simulink model "pid_Modelo"  (R2021b)
settings: Solver=VariableStepAuto  StartTime=0.0  StopTime=1200  RelTol=1e-3
undefined symbols (not defined in the file or in its folder): magnitude, sigbuilder_block
libraries: slpidlib x1
settings Model: Creator=diego  LastModifiedBy=diego
settings SolverCC: AlgebraicLoopSolver=TrustRegion
settings DataIOCC: SaveOutput=off  SaveTime=off  ReturnWorkspaceOutputs=off
settings DebuggingCC: SFMachineParentedDataDiag=warning

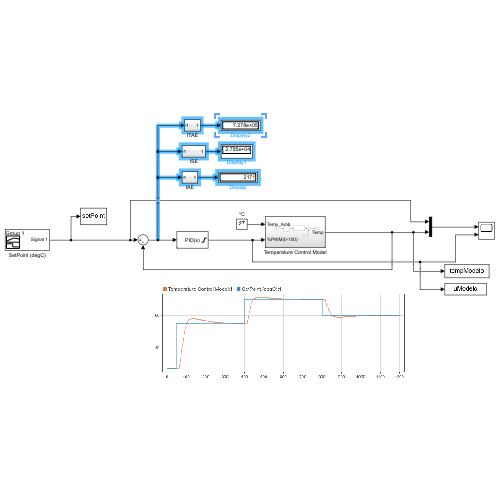
[thumbnail: Simulink's stored preview of the top-level diagram]
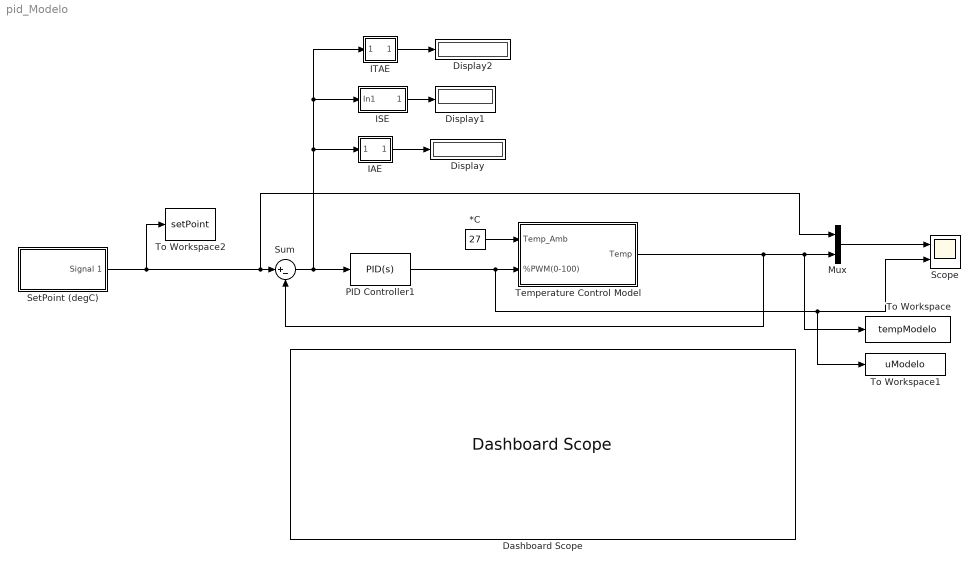
== system pid_Modelo ==
  *C : Constant  Value=27
  Dashboard Scope : DashboardScope  Ymin=23  Ymax=90
  Display : Display
  Display1 : Display
  Display2 : Display
  IAE : Subsystem
  ISE : Subsystem
  ITAE : Subsystem
  Mux : Mux  Inputs=2
  PID Controller1 : slpidlib/PID Controller  Controller=PID  Form=Parallel  TimeDomain=Continuous-time  UseExternalTs=off  SampleTime=-1  IntegratorMethod=Forward Euler  FilterMethod=Forward Euler  ControllerParametersSource=internal  P=3.58266232285661  I=0.0448736690379743  D=10.3284593159219  UseFilter=on  N=0.0959425813529886  TunerSelectOption=Transfer Function Based (PID Tuner App)  InitialConditionSource=internal  InitialConditionForIntegrator=0  InitialConditionForFilter=0  DifferentiatorICPrevScaledInput=0  ExternalReset=none  TrackingMode=off  Kt=1  LimitOutput=on  SatLimitsSource=internal  UpperSaturationLimit=100  LowerSaturationLimit=0  LinearizeAsGain=on  AntiWindupMode=none  Kb=1  POutMin=[]  POutMax=[]  IOutMin=[]  IOutMax=[]  DOutMin=[]  DOutMax=[]  NOutMin=[]  NOutMax=[]  SumOutMin=[]  SumOutMax=[]  SaturationOutMin=[]  SaturationOutMax=[]  PParamMin=[]  PParamMax=[]  IParamMin=[]  IParamMax=[]  DParamMin=[]  DParamMax=[]  NParamMin=[]  NParamMax=[]  KbParamMin=[]  KbParamMax=[]  KtParamMin=[]  KtParamMax=[]  KbOutMin=[]  KbOutMax=[]  KtOutMin=[]  KtOutMax=[]  IntegratorOutMin=[]  IntegratorOutMax=[]  FilterOutMin=[]  FilterOutMax=[]  SumI1OutMin=[]  SumI1OutMax=[]  SumI2OutMin=[]  SumI2OutMax=[]  SumI3OutMin=[]  SumI3OutMax=[]  SumI4OutMin=[]  SumI4OutMax=[]  SumDOutMin=[]  SumDOutMax=[]  DifferentiatorOutMin=[]  DifferentiatorOutMax=[]  FilterDiffOutCoefMin=[]  FilterDiffOutCoefMax=[]  ReciprocalOutMin=[]  ReciprocalOutMax=[]  SumDenOutMin=[]  SumDenOutMax=[]  SumNumOutMin=[]  SumNumOutMax=[]  DivideOutMin=[]  DivideOutMax=[]  UdiffTsProdOutMin=[]  UdiffTsProdOutMax=[]  NTsProdOutMin=[]  NTsProdOutMax=[]  UintegralTsProdOutMin=[]  UintegralTsProdOutMax=[]  UngainTsProdOutMin=[]  UngainTsProdOutMax=[]  IntegratorContinuousStateAttributes=''  IntegratorStateMustResolveToSignalObject=off  IntegratorRTWStateStorageClass=Auto  FilterContinuousStateAttributes=''  FilterStateMustResolveToSignalObject=off  FilterRTWStateStorageClass=Auto  ParallelPVariant=InternalParameters  IdealPVariant=Disabled  IVariant=InternalParameters  DVariant=InternalParameters  IntegratorVariant=Continuous  SatVariant=Enabled  AWVariant=Passthrough  PCopyVariant=Disabled  TRVariant=Disabled  FdbkBlocksVariant=Forward  IdealPFdbkVariant=Disabled  SatFdbkVariant=Disabled  DerivativeFilterVariant=ContFilter  NVariant=InternalParameters  NCopyVariant=Disabled  FilterICVariant=InternalICsFilter  IntegratorICVariant=InternalICs  ExternalResetVariant=Disabled  TRSumVariant=Passthrough  SumFdbkVariant=Disabled  SumVariant=Sum_PID  TsampFilterVariant=InternalTs  TsampNgainVariant=Passthrough  TsampIntegralVariant=Passthrough  ExternalSaturationOutDataTypeStr=Inherit: Same as second input
  Scope : Scope  NumInputPorts=2
  SetPoint (degC) : Subsystem  Tag=STV Subsys  LoadFcn=sigbuilder_block('load');  StartFcn=sigbuilder_block('start');  StopFcn=sigbuilder_block('stop');  ClipboardFcn=sigbuilder_block('clipboard');  mask(Sigbuilder block){tuvar=[0:10]}
      mask help: Simulink:masks:SigbuilderBlock_MD
      mask init:
      | if ~strcmp(get_param(bdroot(gcbh),'SimulationStatus'),'stopped') tuvar = sigbuilder_block('maskInit'); end
      settings: CopyFcn=sigbuilder_block('copy');  DeleteFcn=sigbuilder_block('delete');  ModelCloseFcn=sigbuilder_block('modelClose');  PreSaveFcn=sigbuilder_block('preSave');  PauseFcn=sigbuilder_block('pause');  ContinueFcn=sigbuilder_block('continue');  NameChangeFcn=sigbuilder_block('namechange');  OpenFcn=sigbuilder_block('open',[53.4 0 1093.2 552.6 ]);  CloseFcn=sigbuilder_block('close');
      mask Display: plot(0, 0, 100, 100,[2, 2, 32, 32, 2], [68, 8, 8, 68, 68],[32, 2], [38, 38], [32, 19, 2],[53, 60, 44], [32, 17, 17, 2],[16, 16, 31, 31]);txt = getActiveGroup(gcbh);text(2, 100, txt,'verticalAlignment', 'top');
  Sum : Sum  Inputs=|+-
  Temperature Control Model : Subsystem
  To Workspace : ToWorkspace  VariableName=tempModelo  SampleTime=1
      settings: Save2DSignal=2-D array (concatenate along first dimension)
  To Workspace1 : ToWorkspace  VariableName=uModelo  SampleTime=1
      settings: Save2DSignal=2-D array (concatenate along first dimension)
  To Workspace2 : ToWorkspace  VariableName=setPoint  SampleTime=1
      settings: Save2DSignal=2-D array (concatenate along first dimension)
  wires:
  SetPoint (degC)/1(Signal 1) -> To Workspace2/1, Mux/1, Sum/1
  Sum/1 -> ITAE/1(In1), ISE/1(In1), IAE/1(In1), PID Controller1/1
  *C/1 -> Temperature Control Model/1(Temp_Amb)
  PID Controller1/1 -> To Workspace1/1, Scope/2, Temperature Control Model/2(%PWM(0-100))
  Mux/1 -> Scope/1
  Temperature Control Model/1(Temp) -> Sum/2, To Workspace/1, Mux/2
  IAE/1(Out1) -> Display/1
  ITAE/1(Out1) -> Display2/1
  ISE/1(Out1) -> Display1/1

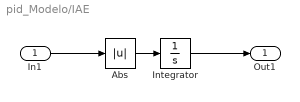
== system pid_Modelo/IAE ==
  In1 : Inport
  Abs : Abs
  Integrator : Integrator
  Out1 : Outport
  wires:
  Abs/1 -> Integrator/1
  In1/1 -> Abs/1
  Integrator/1 -> Out1/1

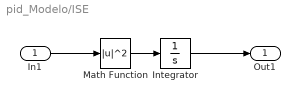
== system pid_Modelo/ISE ==
  In1 : Inport
  Integrator : Integrator
  Math Function : Math  Operator=magnitude^2  SaturateOnIntegerOverflow=on
  Out1 : Outport
  wires:
  Integrator/1 -> Out1/1
  In1/1 -> Math Function/1
  Math Function/1 -> Integrator/1

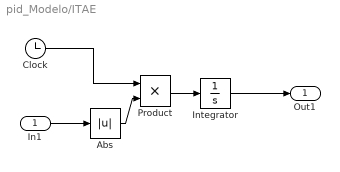
== system pid_Modelo/ITAE ==
  In1 : Inport
  Abs : Abs
  Clock : Clock
  Integrator : Integrator
  Product : Product
  Out1 : Outport
  wires:
  Integrator/1 -> Out1/1
  Product/1 -> Integrator/1
  In1/1 -> Abs/1
  Clock/1 -> Product/1
  Abs/1 -> Product/2

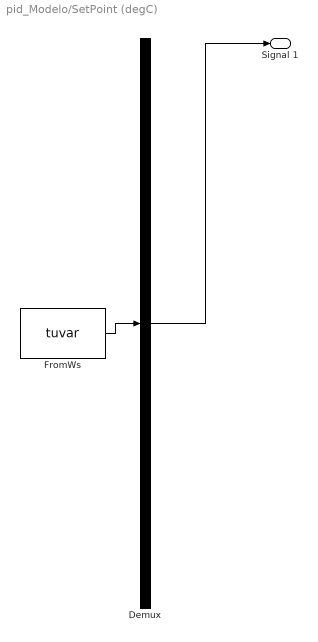
== system pid_Modelo/SetPoint (degC) ==
  Demux : Demux  Tag=STV Demux  Outputs=1
      settings: DisplayOption=none
  FromWs : FromWorkspace  Tag=STV FromWs  VariableName=tuvar
      SigBuilderData=|
      | common.afterFinalStr = 'Extrapolate'
      | common.sampleTime = 0
      | dataSet.timeRange = [0 1200]
      | dataSet.name = 'Group 1'
      | sbobj.Groups.Name = 'Group 1'
      | sbobj.Groups.Signals.Name = 'Signal 1'
      | sbobj.Groups.Signals.XData = [0 50 50 400 400 800 800 1200]
      | sbobj.Groups.Signals.YData = [27 27 55 55 70.1 70.1 60 60]
      | sbobj.Groups.TimeRange = [0 1200]
  Signal 1 : Outport  Tag=STV Outport
  wires:
  Demux/1 -> Signal 1/1
  FromWs/1 -> Demux/1

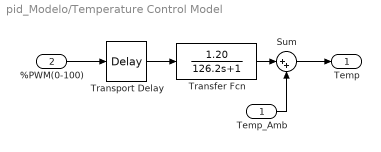
== system pid_Modelo/Temperature Control Model ==
  Temp_Amb : Inport
  %PWM(0-100) : Inport  Port=2
  Sum : Sum  Inputs=|++
  Transfer Fcn : TransferFcn  Numerator=[1.20]  Denominator=[126.2, 1]
  Transport Delay : TransportDelay  DelayTime=14.23
  Temp : Outport
  wires:
  Transport Delay/1 -> Transfer Fcn/1
  Temp_Amb/1 -> Sum/2
  Sum/1 -> Temp/1
  Transfer Fcn/1 -> Sum/1
  %PWM(0-100)/1 -> Transport Delay/1
